simulink model "srotut1"  (Simulink 6.0)
settings: Solver=ode45  SolverMode=SingleTasking  StartTime=0.0  StopTime=50  RelTol=1e-3  AbsTol=1e-6
PreLoadFcn:
  | srotut1_dat
undefined symbols (not defined in the file or in its folder): Kint, w0, zeta
libraries: srolib x1
settings Model: Creator=lparsons  LastModifiedBy=lparsons  ExtModeTrigMode=oneshot
settings DataIOCC: LimitDataPoints=off  SaveState=on  StateSaveName=x  TimeSaveName=t  OutputSaveName=y  SignalLoggingName=DataLog
settings OptimizationCC: BooleanDataType=off
settings DebuggingCC: ConsistencyChecking=warning  CheckExecutionContextPreStartOutputMsg=on  CheckExecutionContextRuntimeOutputMsg=on  SolverPrmCheckMsg=none
settings HardwareCC: TargetUnknown=on
settings ModelReferenceCC: UpdateModelReferenceTargets=IfOutOfDate
settings GRTTargetCC: LifeSpan=inf
settings SFSimCC: SFSimApplyToAllLibs=on  SFSimBuildMode=Incremental

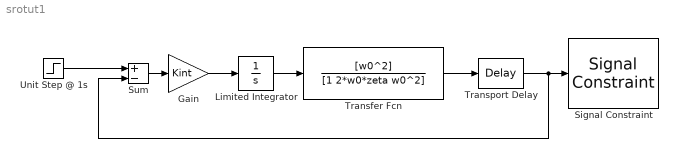
== system srotut1 ==
  Gain : Gain  Gain=Kint  SaturateOnIntegerOverflow=on
  Limited Integrator : Integrator  LimitOutput=on  UpperSaturationLimit=1.5  LowerSaturationLimit=-1.5
  Signal Constraint : srolib/Signal Constraint  Tag=sro_block  DialogPosition=[0.1 0.25 0.45 0.31]  SaveIn=workspace
  Sum : Sum  Inputs=+-  SaturateOnIntegerOverflow=on  InputSameDT=on
  Transfer Fcn : TransferFcn  Numerator=[w0^2]  Denominator=[1 2*w0*zeta w0^2]
  Transport Delay : TransportDelay
  Unit Step @ 1s : Step  SampleTime=0
  wires:
  Transport Delay/1 -> Sum/2, Signal Constraint/1
  Transfer Fcn/1 -> Transport Delay/1
  Limited Integrator/1 -> Transfer Fcn/1
  Gain/1 -> Limited Integrator/1
  Sum/1 -> Gain/1
  Unit Step @ 1s/1 -> Sum/1
